simulink model "control_sist_no_lineal_meto_ganancias"  (R2016a)
settings: Solver=VariableStepAuto  StartTime=0.0  StopTime=10  RelTol=1e-3
settings Model: Creator=Daniel  LastModifiedBy=Daniel

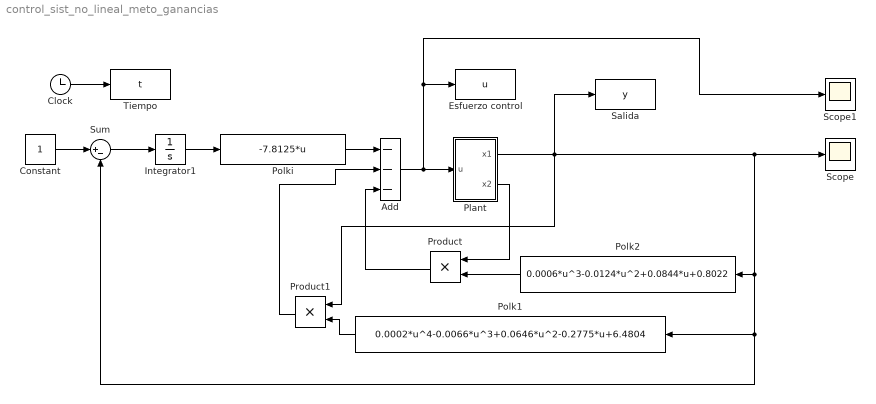
== system control_sist_no_lineal_meto_ganancias ==
  Add : Sum  Inputs=---
  Clock : Clock
  Constant : Constant
  Esfuerzo control : ToWorkspace  VariableName=u  SaveFormat=Timeseries  SampleTime=-1
  Integrator1 : Integrator
  Plant : Subsystem
  Polk1 : Fcn  Expr=0.0002*u^4-0.0066*u^3+0.0646*u^2-0.2775*u+6.4804
  Polk2 : Fcn  Expr=0.0006*u^3-0.0124*u^2+0.0844*u+0.8022
  Polki : Fcn  Expr=-7.8125*u
  Product : Product
  Product1 : Product
  Salida : ToWorkspace  VariableName=y  SaveFormat=Timeseries  SampleTime=-1
  Scope : Scope
  Scope1 : Scope
  Sum : Sum  Inputs=|+-
  Tiempo : ToWorkspace  VariableName=t  SaveFormat=Timeseries  SampleTime=-1
  wires:
  Plant/1(x1) -> Product1/1, Salida/1, Polk1/1, Sum/2, Polk2/1, Scope/1
  Add/1 -> Esfuerzo control/1, Scope1/1, Plant/1(u)
  Product/1 -> Add/3
  Plant/2(x2) -> Product/1
  Polk1/1 -> Product1/2
  Polk2/1 -> Product/2
  Integrator1/1 -> Polki/1
  Polki/1 -> Add/1
  Sum/1 -> Integrator1/1
  Constant/1 -> Sum/1
  Clock/1 -> Tiempo/1
  Product1/1 -> Add/2

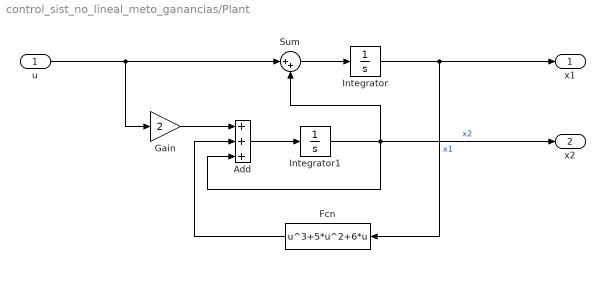
== system control_sist_no_lineal_meto_ganancias/Plant ==
  u : Inport
  Add : Sum  Inputs=+++
  Fcn : Fcn  Expr=u^3+5*u^2+6*u
  Gain : Gain  Gain=2
  Integrator : Integrator
  Integrator1 : Integrator
  Sum : Sum  Inputs=|++
  x1 : Outport
  x2 : Outport  Port=2
  wires:
  Add/1 -> Integrator1/1
  Sum/1 -> Integrator/1
  Integrator1/1 -> x2/1, Add/3, Sum/2  "x2"
  Gain/1 -> Add/1
  Fcn/1 -> Add/2
  Integrator/1 -> x1/1, Fcn/1  "x1"
  u/1 -> Gain/1, Sum/1
